simulink model "StateObserverTest4"  (R2018b)
settings: Solver=VariableStepAuto  StartTime=0.0  StopTime=30  RelTol=1e-3
values from neighbouring files (symbols this model uses):
  GdSpeed = c2d(Gspeed,Ts,'tustin')    [DiscreteObserverAndSFB.m]
  Ts = 0.01    [DiscreteObserverAndSFB.m]
undefined symbols (not defined in the file or in its folder): DiscIntNeverNeededParam
settings Model: Creator=Yahya  LastModifiedBy=Yahya

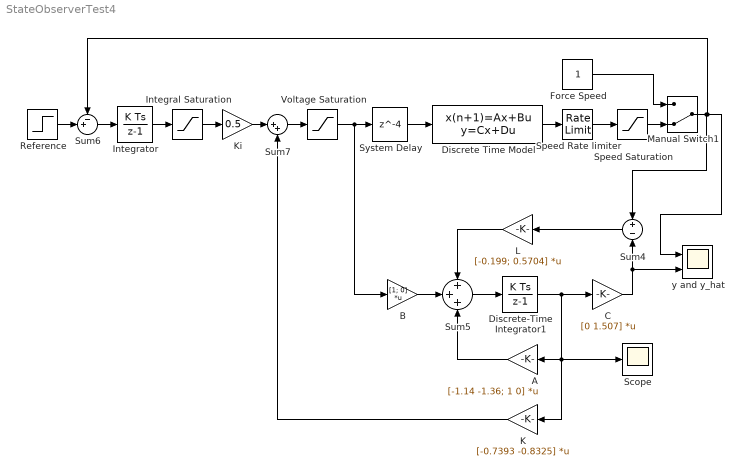
== system StateObserverTest4 ==
  A : Gain  Gain=[-1.14 -1.36; 1 0]  Multiplication=Matrix(K*u)
  B : Gain  Gain=[1; 0]  Multiplication=Matrix(K*u)
  C : Gain  Gain=[0 1.507]  Multiplication=Matrix(K*u)
  Discrete Time Model : DiscreteStateSpace  A=GdSpeed.A  B=GdSpeed.B  C=GdSpeed.C  D=0  SampleTime=Ts
  Discrete-Time Integrator1 : DiscreteIntegrator  SampleTime=Ts  ICPrevOutput=DiscIntNeverNeededParam  ICPrevScaledInput=DiscIntNeverNeededParam
  Force Speed : Constant
  Integral Saturation : Saturate  UpperLimit=5/0.5  LowerLimit=-5/0.5
  Integrator : DiscreteIntegrator  SampleTime=Ts  ICPrevOutput=DiscIntNeverNeededParam  ICPrevScaledInput=DiscIntNeverNeededParam
  K : Gain  Gain=[-0.7393 -0.8325]  Multiplication=Matrix(K*u)
  Ki : Gain  Gain=0.5
  L : Gain  Gain=[-0.199; 0.5704]  Multiplication=Matrix(K*u)
  Manual Switch1 : ManualSwitch  CurrentSetting=0
  Reference : Step  SampleTime=0
  Scope : Scope
  Speed Rate limiter : RateLimiter  RisingSlewLimit=0.65  FallingSlewLimit=-0.65  SampleTimeMode=inherited
  Speed Saturation : Saturate  UpperLimit=1000  LowerLimit=0
  Sum4 : Sum  Inputs=+-
  Sum5 : Sum  Inputs=+++
  Sum6 : Sum  Inputs=-+|
  Sum7 : Sum  Inputs=|++
  System Delay : Delay  DelayLength=4  SampleTime=Ts
  Voltage Saturation : Saturate  UpperLimit=5  LowerLimit=0
  y and y_hat : Scope  NumInputPorts=2
  wires:
  System Delay/1 -> Discrete Time Model/1
  Sum7/1 -> Voltage Saturation/1
  C/1 -> Sum4/2, y and y_hat/2
  Force Speed/1 -> Manual Switch1/1
  Discrete Time Model/1 -> Speed Rate limiter/1
  Ki/1 -> Sum7/1
  Reference/1 -> Sum6/2
  K/1 -> Sum7/2
  Sum4/1 -> L/1
  Discrete-Time Integrator1/1 -> C/1, Scope/1, A/1, K/1
  L/1 -> Sum5/1
  Speed Rate limiter/1 -> Speed Saturation/1
  Voltage Saturation/1 -> System Delay/1, B/1
  Sum5/1 -> Discrete-Time Integrator1/1
  B/1 -> Sum5/2
  A/1 -> Sum5/3
  Speed Saturation/1 -> Manual Switch1/2
  Sum6/1 -> Integrator/1
  Integrator/1 -> Integral Saturation/1
  Integral Saturation/1 -> Ki/1
  Manual Switch1/1 -> y and y_hat/1, Sum6/1, Sum4/1
